simulink model "SnapshotPlanner"  (R2024b)
settings: Solver=FixedStepAuto  StartTime=0.0  StopTime=10.0  RelTol=1e-3  EnableMultiTasking=on
values from neighbouring files (symbols this model uses):
  timeResolution = 0.1    [helperSLHighwayLaneChangePlannerSetup.m]
undefined symbols (not defined in the file or in its folder): actorProfiles, computeMethod
settings Model: Creator=The MathWorks, Inc.  LastModifiedBy=grape
settings SolverCC: AlgebraicLoopSolver=TrustRegion  MaxZcPerStep=1
settings DataIOCC: SaveOutput=off
settings OptimizationCC: DefaultParameterBehavior=Inlined  InlineInvariantSignals=on  EnhancedBackFolding=on  PassReuseOutputArgsAs=Individual arguments  ZeroExternalMemoryAtStartup=off  ZeroInternalMemoryAtStartup=off  EfficientFloat2IntCast=on  OptimizeBlockOrder=speed  DifferentSizesBufferReuse=on  OptimizationCustomize=off  EfficientTunableParamExpr=on
settings DebuggingCC: ParameterTunabilityLossMsg=error  UnconnectedInputMsg=warning  UnconnectedOutputMsg=warning  UnconnectedLineMsg=warning  ModelReferenceSymbolNameMessage=none  SubsystemReferenceDiagnosticForUnitTest=warning
settings HardwareCC: ProdLongLongMode=on
settings ModelReferenceCC: EnableRefExpFcnMdlSchedulingChecks=on  ModelReferenceNumInstancesAllowed=Single  PropagateVarSize=During execution
settings RTWCC: Description=Embedded Coder  SystemTargetFile=ert.tlc  TemplateMakefile=ert_default_tmf  RTWVerbose=off  BuildConfiguration=Faster Runs  PortableWordSizes=on  CodeExecutionProfiling=on  CodeProfilingSaveOptions=AllData  TargetLang=C++  GPUComputeCapability=3.5  DLArmComputeVersion=19.05
settings CodeAppCC: ForceParamTrailComments=on  IgnoreCustomStorageClasses=off  OperatorAnnotations=on  SimulinkDataObjDesc=on  SFDataObjDesc=on  CustomSymbolStrGlobalVar=$N$M  CustomSymbolStrType=$N$M_T  CustomSymbolStrFcn=APV_$N$M$F  CustomSymbolStrMacro=$N$M  InsertBlockDesc=on
settings ERTTargetCC: TargetLangStandard=C++03 (ISO)  GenerateSampleERTMain=on  CombineSignalStateStructs=on  CodeInterfacePackaging=C++ class  SupportVariableSizeSignals=on  RootIOFormat=Structure reference  ERTCustomFileTemplate=example_file_process.tlc  DynamicArrayContainerType=coder::array

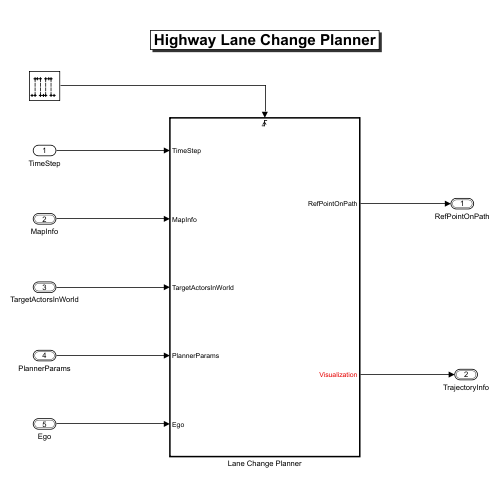
[thumbnail: Simulink's stored preview of the top-level diagram]
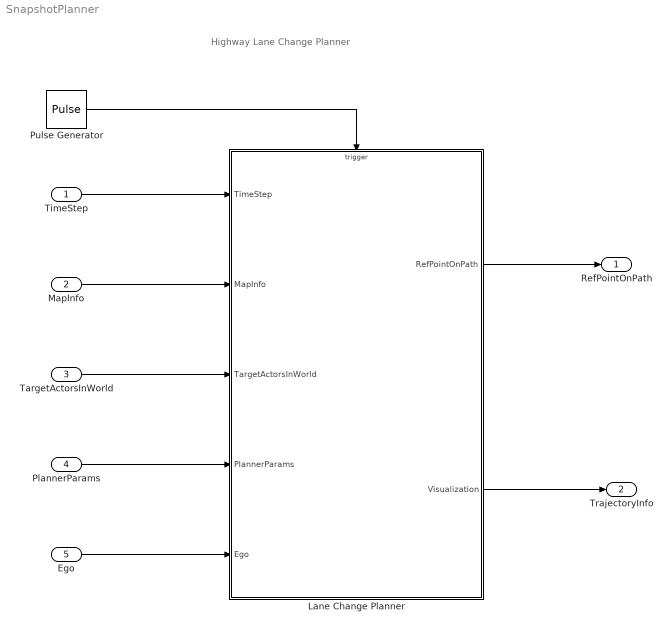
== system SnapshotPlanner ==
  note: Highway Lane Change Planner
  TimeStep : Inport
  MapInfo : Inport  Port=2  OutDataTypeStr=Bus: BusMapInfo  BusOutputAsStruct=on
  TargetActorsInWorld : Inport  Port=3  OutDataTypeStr=Bus: BusActorsEgo  BusOutputAsStruct=on
  PlannerParams : Inport  Port=4  OutDataTypeStr=Bus: BusPlannerParams  BusOutputAsStruct=on
  Ego : Inport  Port=5  OutDataTypeStr=Bus: BusVehiclePose
  Lane Change Planner : Subsystem
  Pulse Generator : DiscretePulseGenerator  SampleTime=timeResolution
  RefPointOnPath : Outport  OutDataTypeStr=Bus: BusRefPointOnPath  BusOutputAsStruct=on
  TrajectoryInfo : Outport  Port=2  OutDataTypeStr=Bus: BusVisualizationInfo  BusOutputAsStruct=on
  wires:
  TimeStep/1 -> Lane Change Planner/1(TimeStep)
  MapInfo/1 -> Lane Change Planner/2(MapInfo)
  TargetActorsInWorld/1 -> Lane Change Planner/3(TargetActorsInWorld)
  PlannerParams/1 -> Lane Change Planner/4(PlannerParams)
  Ego/1 -> Lane Change Planner/5(Ego)
  Lane Change Planner/2(Visualization) -> TrajectoryInfo/1
  Pulse Generator/1 -> Lane Change Planner/Trigger
  Lane Change Planner/1(RefPointOnPath) -> RefPointOnPath/1

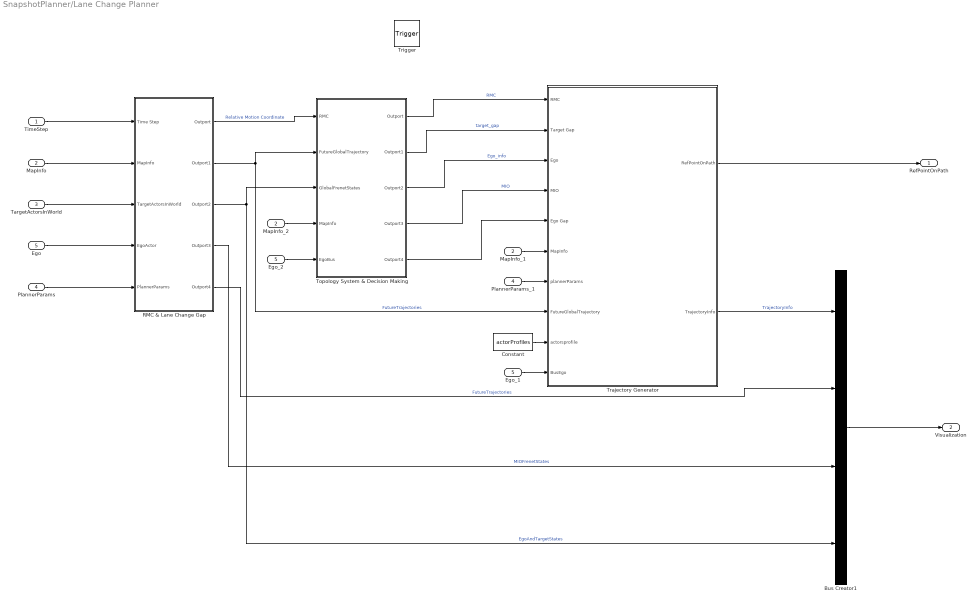
== system SnapshotPlanner/Lane Change Planner ==
  TimeStep : Inport
  MapInfo : Inport  Port=2  OutDataTypeStr=Bus: BusMapInfo  BusOutputAsStruct=on
  TargetActorsInWorld : Inport  Port=3  OutDataTypeStr=Bus: BusActorsEgo  BusOutputAsStruct=on
  PlannerParams : Inport  Port=4  OutDataTypeStr=Bus: BusPlannerParams  BusOutputAsStruct=on
  Ego : Inport  Port=5  OutDataTypeStr=Bus: BusVehiclePose
  Trigger : TriggerPort  VariantControl=(inherit)  InitialTriggerSignalState=zero  PortDimensions=1
  Bus Creator1 : BusCreator  Inputs=4  OutDataTypeStr=Bus: BusVisualizationInfo
  Constant : Constant  Value=actorProfiles  OutDataTypeStr=Bus: BusActorProfiles
  Ego_1 : InportShadow  Port=5  OutDataTypeStr=Bus: BusVehiclePose
  Ego_2 : InportShadow  Port=5  OutDataTypeStr=Bus: BusVehiclePose
  MapInfo_1 : InportShadow  Port=2  OutDataTypeStr=Bus: BusMapInfo  BusOutputAsStruct=on
  MapInfo_2 : InportShadow  Port=2  OutDataTypeStr=Bus: BusMapInfo  BusOutputAsStruct=on
  PlannerParams_1 : InportShadow  Port=4  OutDataTypeStr=Bus: BusPlannerParams  BusOutputAsStruct=on
  "RMC & Lane Change Gap " : Subsystem
  Topology System & Decision Making : Subsystem
  Trajectory Generator : Subsystem
  RefPointOnPath : Outport  OutDataTypeStr=Bus: BusRefPointOnPath  BusOutputAsStruct=on
  Visualization : Outport  Port=2  OutDataTypeStr=Bus: BusVisualizationInfo  BusOutputAsStruct=on
  wires:
  "RMC & Lane Change Gap "/5(Outport4) -> Bus Creator1/2  "FutureTrajectories"
  MapInfo_2/1 -> Topology System & Decision Making/4(MapInfo)
  "RMC & Lane Change Gap "/3(Outport2) -> Bus Creator1/4, Topology System & Decision Making/3(GlobalFrenetStates)  "EgoAndTargetStates"
  "RMC & Lane Change Gap "/1(Outport) -> Topology System & Decision Making/1(RMC)  "Relative Motion Coordinate"
  Topology System & Decision Making/5(Outport4) -> Trajectory Generator/5(Ego Gap)
  Topology System & Decision Making/4(Outport3) -> Trajectory Generator/4(MIO)  "MIO"
  Ego/1 -> "RMC & Lane Change Gap "/4(EgoActor)
  Ego_1/1 -> Trajectory Generator/10(BusEgo)
  "RMC & Lane Change Gap "/2(Outport1) -> Trajectory Generator/8(FutureGlobalTrajectory), Topology System & Decision Making/2(FutureGlobalTrajectory)  "FutureTrajectories"
  PlannerParams/1 -> "RMC & Lane Change Gap "/5(PlannerParams)
  Trajectory Generator/2(TrajectoryInfo) -> Bus Creator1/1  "TrajectoryInfo"
  TimeStep/1 -> "RMC & Lane Change Gap "/1(Time Step)
  TargetActorsInWorld/1 -> "RMC & Lane Change Gap "/3(TargetActorsInWorld)
  Topology System & Decision Making/1(Outport) -> Trajectory Generator/1(RMC)  "RMC"
  Topology System & Decision Making/2(Outport1) -> Trajectory Generator/2(Target Gap)  "target_gap"
  PlannerParams_1/1 -> Trajectory Generator/7(plannerParams)
  MapInfo_1/1 -> Trajectory Generator/6(MapInfo)
  Constant/1 -> Trajectory Generator/9(actorsprofile)
  Topology System & Decision Making/3(Outport2) -> Trajectory Generator/3(Ego)  "Ego_info"
  MapInfo/1 -> "RMC & Lane Change Gap "/2(MapInfo)
  Bus Creator1/1 -> Visualization/1
  "RMC & Lane Change Gap "/4(Outport3) -> Bus Creator1/3  "MIOFrenetStates"
  Ego_2/1 -> Topology System & Decision Making/5(EgoBus)
  Trajectory Generator/1(RefPointOnPath) -> RefPointOnPath/1

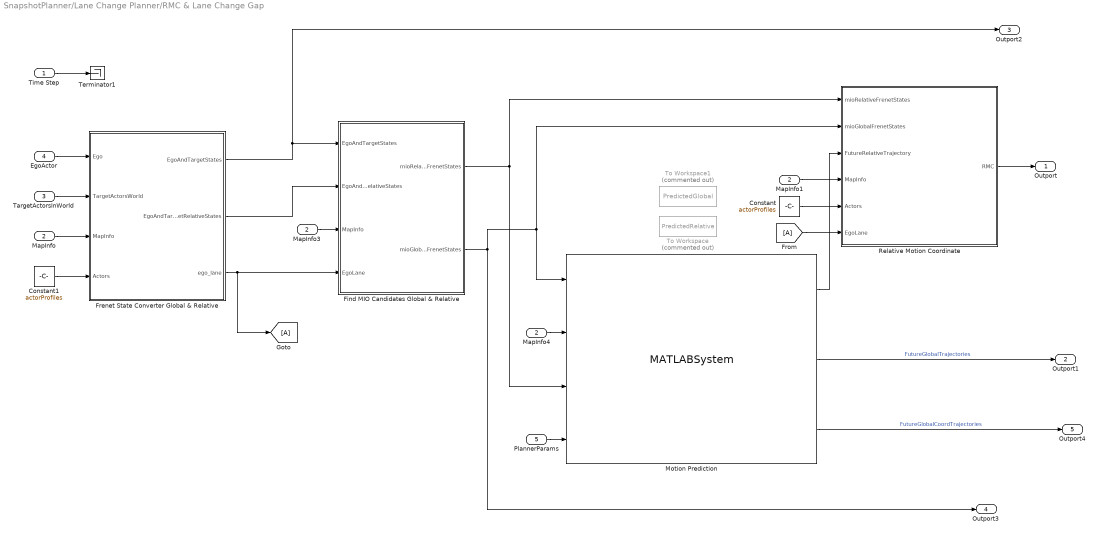
== system SnapshotPlanner/Lane Change Planner/RMC & Lane Change Gap  ==
  Time Step : Inport
  MapInfo : Inport  Port=2  OutDataTypeStr=Bus: BusMapInfo
  TargetActorsInWorld : Inport  Port=3  OutDataTypeStr=Bus: BusActorsEgo
  EgoActor : Inport  Port=4  OutDataTypeStr=Bus: BusVehiclePose
  PlannerParams : Inport  Port=5  OutDataTypeStr=Bus: BusPlannerParams
  Constant : Constant  Value=actorProfiles  OutDataTypeStr=Bus: BusActorProfiles
  Constant1 : Constant  Value=actorProfiles  OutDataTypeStr=Bus: BusActorProfiles
  Find MIO Candidates Global & Relative : MATLAB Function  TreatAsAtomicUnit=on
  Frenet State Converter Global & Relative : MATLAB Function  TreatAsAtomicUnit=on
  From : From
  Goto : Goto
  MapInfo1 : InportShadow  Port=2  OutDataTypeStr=Bus: BusMapInfo
  MapInfo3 : InportShadow  Port=2  OutDataTypeStr=Bus: BusMapInfo
  MapInfo4 : InportShadow  Port=2  OutDataTypeStr=Bus: BusMapInfo
  Motion Prediction : MATLABSystem  System=HelperMotionPrediction_RMC  SimulateUsing=Interpreted execution
      mask Type: HelperMotionPrediction_RMC
      mask Display:
      | disp('HelperMotionPrediction_RMC');
      | port_label('input',1,'MIOs_Global');
      | port_label('input',2,'MapInfo');
      | port_label('input',3,'MIOs_Relative');
      | port_label('input',4,'Params');
      | port_label('output',1,'FutureRelativeTrajectories');
      | port_label('output',2,'FutureGlobalTrajectories');
      | port_label('output',3,'FutureGlobalCoordTrajectories');
  Relative Motion Coordinate : MATLAB Function  TreatAsAtomicUnit=on
  Terminator1 : Terminator
  To Workspace : ToWorkspace  Commented=on  VariableName=PredictedRelative  SaveFormat=Timeseries  SampleTime=-1
  To Workspace1 : ToWorkspace  Commented=on  VariableName=PredictedGlobal  SaveFormat=Timeseries  SampleTime=-1
  Outport : Outport  OutDataTypeStr=Bus: BusRelativeMotionCoordinate
  Outport1 : Outport  Port=2  OutDataTypeStr=Bus: BusPredictedTrajectories
  Outport2 : Outport  Port=3  OutDataTypeStr=Bus: BusEgoAndTargetStates
  Outport3 : Outport  Port=4  OutDataTypeStr=Bus: BusMIOFrenetStates
  Outport4 : Outport  Port=5
  wires:
  Frenet State Converter Global & Relative/1(EgoAndTargetStates) -> Outport2/1, Find MIO Candidates Global & Relative/1(EgoAndTargetStates)
  Time Step/1 -> Terminator1/1
  EgoActor/1 -> Frenet State Converter Global & Relative/1(Ego)
  TargetActorsInWorld/1 -> Frenet State Converter Global & Relative/2(TargetActorsWorld)
  MapInfo/1 -> Frenet State Converter Global & Relative/3(MapInfo)
  Frenet State Converter Global & Relative/2(EgoAndTargetRelativeStates) -> Find MIO Candidates Global & Relative/2(EgoAndTargetRelativeStates)
  MapInfo3/1 -> Find MIO Candidates Global & Relative/3(MapInfo)
  Find MIO Candidates Global & Relative/1(mioRelativeFrenetStates) -> Relative Motion Coordinate/1(mioRelativeFrenetStates), Motion Prediction/3
  MapInfo4/1 -> Motion Prediction/2
  PlannerParams/1 -> Motion Prediction/4
  Find MIO Candidates Global & Relative/2(mioGlobalFrenetStates) -> Relative Motion Coordinate/2(mioGlobalFrenetStates), Motion Prediction/1, Outport3/1
  Motion Prediction/1 -> Relative Motion Coordinate/3(FutureRelativeTrajectory)
  Relative Motion Coordinate/1(RMC) -> Outport/1
  Motion Prediction/2 -> Outport1/1  "FutureGlobalTrajectories"
  MapInfo1/1 -> Relative Motion Coordinate/4(MapInfo)
  Constant/1 -> Relative Motion Coordinate/5(Actors)
  Motion Prediction/3 -> Outport4/1  "FutureGlobalCoordTrajectories"
  Constant1/1 -> Frenet State Converter Global & Relative/4(Actors)
  Frenet State Converter Global & Relative/3(ego_lane) -> Find MIO Candidates Global & Relative/4(EgoLane), Goto/1
  From/1 -> Relative Motion Coordinate/6(EgoLane)

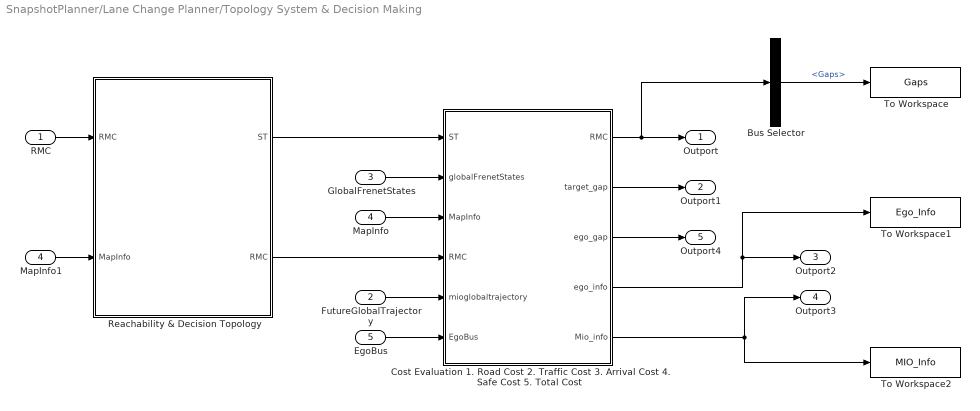
== system SnapshotPlanner/Lane Change Planner/Topology System & Decision Making ==
  RMC : Inport  OutDataTypeStr=Bus: BusRelativeMotionCoordinate
  FutureGlobalTrajectory : Inport  Port=2
  GlobalFrenetStates : Inport  Port=3  OutDataTypeStr=Bus: BusEgoAndTargetStates
  MapInfo : Inport  Port=4
  EgoBus : Inport  Port=5
  Bus Selector : BusSelector  OutputSignals=Gaps
  Cost Evaluation 1. Road Cost 2. Traffic Cost 3. Arrival Cost 4. Safe Cost 5. Total Cost : MATLAB Function  TreatAsAtomicUnit=on
  MapInfo1 : InportShadow  Port=4
  Reachability & Decision Topology : MATLAB Function  TreatAsAtomicUnit=on
  To Workspace : ToWorkspace  VariableName=Gaps  SaveFormat=Timeseries  SampleTime=-1
  To Workspace1 : ToWorkspace  VariableName=Ego_Info  SampleTime=-1
  To Workspace2 : ToWorkspace  VariableName=MIO_Info  SampleTime=-1
  Outport : Outport
  Outport1 : Outport  Port=2
  Outport2 : Outport  Port=3
  Outport3 : Outport  Port=4
  Outport4 : Outport  Port=5
  wires:
  Reachability & Decision Topology/2(RMC) -> Cost Evaluation 1. Road Cost 2. Traffic Cost 3. Arrival Cost 4. Safe Cost 5. Total Cost/4("RMC ")
  Reachability & Decision Topology/1(ST) -> Cost Evaluation 1. Road Cost 2. Traffic Cost 3. Arrival Cost 4. Safe Cost 5. Total Cost/1(ST)
  MapInfo/1 -> Cost Evaluation 1. Road Cost 2. Traffic Cost 3. Arrival Cost 4. Safe Cost 5. Total Cost/3(MapInfo)
  FutureGlobalTrajectory/1 -> Cost Evaluation 1. Road Cost 2. Traffic Cost 3. Arrival Cost 4. Safe Cost 5. Total Cost/5(mioglobaltrajectory)
  RMC/1 -> Reachability & Decision Topology/1("RMC ")
  GlobalFrenetStates/1 -> Cost Evaluation 1. Road Cost 2. Traffic Cost 3. Arrival Cost 4. Safe Cost 5. Total Cost/2(globalFrenetStates)
  Cost Evaluation 1. Road Cost 2. Traffic Cost 3. Arrival Cost 4. Safe Cost 5. Total Cost/1(RMC) -> Bus Selector/1, Outport/1
  Cost Evaluation 1. Road Cost 2. Traffic Cost 3. Arrival Cost 4. Safe Cost 5. Total Cost/4(ego_info) -> To Workspace1/1, Outport2/1
  Cost Evaluation 1. Road Cost 2. Traffic Cost 3. Arrival Cost 4. Safe Cost 5. Total Cost/2(target_gap) -> Outport1/1
  Cost Evaluation 1. Road Cost 2. Traffic Cost 3. Arrival Cost 4. Safe Cost 5. Total Cost/5(Mio_info) -> Outport3/1, To Workspace2/1
  Cost Evaluation 1. Road Cost 2. Traffic Cost 3. Arrival Cost 4. Safe Cost 5. Total Cost/3(ego_gap) -> Outport4/1
  Bus Selector/1 -> To Workspace/1  "<Gaps>"
  MapInfo1/1 -> Reachability & Decision Topology/2(MapInfo)
  EgoBus/1 -> Cost Evaluation 1. Road Cost 2. Traffic Cost 3. Arrival Cost 4. Safe Cost 5. Total Cost/6(EgoBus)

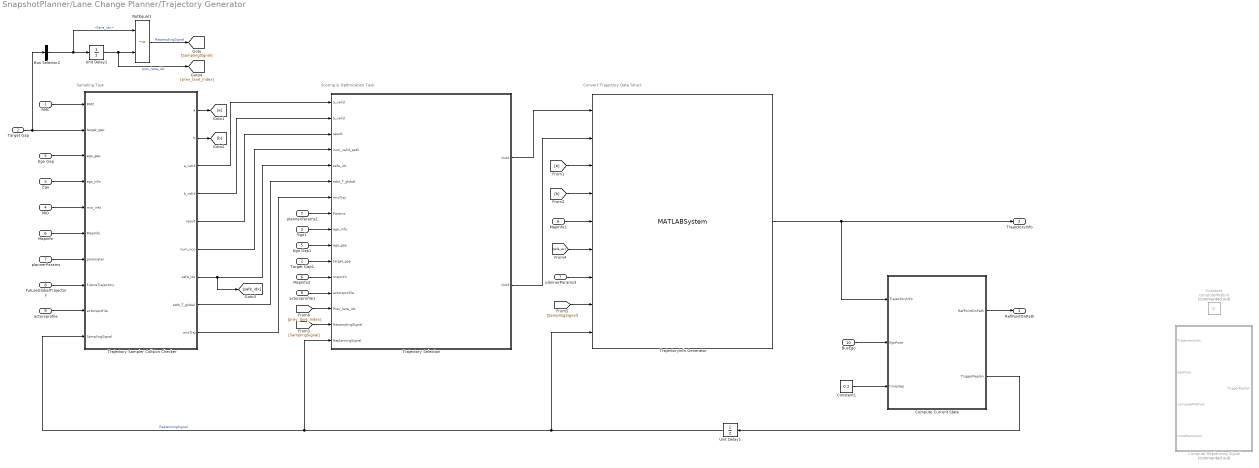
== system SnapshotPlanner/Lane Change Planner/Trajectory Generator ==
  note: Convert Trajectory Data Struct
  note: Scoring & Optimization Task
  note: Sampling Task
  RMC : Inport  OutDataTypeStr=Bus: BusRelativeMotionCoordinate
  Target Gap : Inport  Port=2
  Ego : Inport  Port=3
  MIO : Inport  Port=4
  Ego Gap : Inport  Port=5
  MapInfo : Inport  Port=6
  plannerParams : Inport  Port=7
  FutureGlobalTrajectory : Inport  Port=8
  actorsprofile : Inport  Port=9
  BusEgo : Inport  Port=10  OutDataTypeStr=Bus: BusVehiclePose
  Bus Selector2 : BusSelector  OutputSignals=lane_idx
  Compute Current State : MATLAB Function  TreatAsAtomicUnit=on
  Compute Replanning Signal : MATLAB Function  Commented=on  TreatAsAtomicUnit=on
  Constant : Constant  Commented=on  Value=computeMethod
  Constant1 : Constant  Value=0.2
  Ego Gap1 : InportShadow  Port=5
  Ego1 : InportShadow  Port=3
  MapInfo1 : InportShadow  Port=6
  MapInfo2 : InportShadow  Port=6
  NotEqual1 : RelationalOperator  Operator=~=  OutDataTypeStr=boolean  RndMeth=Simplest  InputSameDT=off
  Target Gap1 : InportShadow  Port=2
  Trajectory Selection : Subsystem  TreatAsAtomicUnit=on
  Trajectory Sampler Collsion Checker : MATLAB Function  TreatAsAtomicUnit=on
  TrajectoryInfo Generator : MATLABSystem  System=HelperMakeTrajectoryInfo  SimulateUsing=Interpreted execution
      mask Type: HelperMakeTrajectoryInfo
      mask Display:
      | disp('HelperMakeTrajectoryInfo');
      | port_label('input',1,'optimal_a');
      | port_label('input',2,'optimal_b');
      | port_label('input',3,'a');
      | port_label('input',4,'b');
      | port_label('input',5,'MapInfo');
      | port_label('input',6,'safe_idx');
      | port_label('input',7,'params');
      | port_label('input',8,'resamplingSignal');
      | port_label('input',9,'replanningSignal');
      | port_label('output',1,'GlobalTrajectories');
  Unit Delay1 : UnitDelay  InitialCondition=true  SampleTime=-1  HasFrameUpgradeWarning=on
  Unit Delay2 : UnitDelay  SampleTime=-1  HasFrameUpgradeWarning=on
  actorsprofile1 : InportShadow  Port=9
  plannerParams1 : InportShadow  Port=7
  plannerParams3 : InportShadow  Port=7
  RefPointOnPath : Outport  OutDataTypeStr=Bus: BusRefPointOnPath
  TrajectoryInfo : Outport  Port=2  OutDataTypeStr=Bus: BusGlobalTrajectories
  wires:
  MapInfo/1 -> Trajectory Sampler Collsion Checker/6(MapInfo)
  Ego/1 -> Trajectory Sampler Collsion Checker/4(ego_info)
  RMC/1 -> Trajectory Sampler Collsion Checker/1(RMC)
  MIO/1 -> Trajectory Sampler Collsion Checker/5(mio_info)
  plannerParams/1 -> Trajectory Sampler Collsion Checker/7(parameter)
  FutureGlobalTrajectory/1 -> Trajectory Sampler Collsion Checker/8(FutureTrajectory)
  actorsprofile/1 -> Trajectory Sampler Collsion Checker/9(actorsprofile)
  Ego Gap/1 -> Trajectory Sampler Collsion Checker/3(ego_gap)
  TrajectoryInfo Generator/1 -> Compute Current State/1(TrajectoryInfo), TrajectoryInfo/1
  Bus Selector2/1 -> NotEqual1/1, Unit Delay2/1  "<lane_idx>"
  Unit Delay2/1 -> [prev_lane_index], NotEqual1/2  "prev_lane_idx"
  Target Gap/1 -> Bus Selector2/1, Trajectory Sampler Collsion Checker/2(target_gap)
  Unit Delay1/1 -> Trajectory Sampler Collsion Checker/10(SamplingSignal), Trajectory Selection/16(ReplanningSignal), TrajectoryInfo Generator/9  "ReplanningSignal"
  NotEqual1/1 -> [SamplingSignal]  "ResamplingSignal"
  Trajectory Sampler Collsion Checker/2(b) -> [b]
  Trajectory Sampler Collsion Checker/1(a) -> [a]
  [a] -> TrajectoryInfo Generator/3
  [b] -> TrajectoryInfo Generator/4
  Trajectory Selection/1(Out2) -> TrajectoryInfo Generator/1
  Trajectory Selection/2(Out3) -> TrajectoryInfo Generator/2
  MapInfo1/1 -> TrajectoryInfo Generator/5
  Trajectory Sampler Collsion Checker/3(a_valid) -> Trajectory Selection/1(a_valid)
  Trajectory Sampler Collsion Checker/4(b_valid) -> Trajectory Selection/2(b_valid)
  Trajectory Sampler Collsion Checker/5(result) -> Trajectory Selection/3(result)
  Trajectory Sampler Collsion Checker/6(num_ncp) -> Trajectory Selection/4(num_valid_path)
  Trajectory Sampler Collsion Checker/7(safe_idx) -> [safe_idx], Trajectory Selection/5(safe_idx)
  Trajectory Sampler Collsion Checker/8(sdot_T_global) -> Trajectory Selection/6(sdot_T_global)
  Trajectory Sampler Collsion Checker/9(mioTraj) -> Trajectory Selection/7(mioTraj)
  plannerParams1/1 -> Trajectory Selection/8(Params)
  Ego1/1 -> Trajectory Selection/9(ego_info)
  Ego Gap1/1 -> Trajectory Selection/10(ego_gap)
  Target Gap1/1 -> Trajectory Selection/11(target_gap)
  MapInfo2/1 -> Trajectory Selection/12(mapinfo)
  actorsprofile1/1 -> Trajectory Selection/13(actorsprofile)
  [safe_idx] -> TrajectoryInfo Generator/6
  plannerParams3/1 -> TrajectoryInfo Generator/7
  [SamplingSignal] -> TrajectoryInfo Generator/8
  [SamplingSignal] -> Trajectory Selection/15(ResamplingSignal)
  [prev_lane_index] -> Trajectory Selection/14(Prev_lane_idx)
  Compute Current State/2(TriggerReplan) -> Unit Delay1/1
  BusEgo/1 -> Compute Current State/2(EgoPose)
  Constant1/1 -> Compute Current State/3(timestep)
  Compute Current State/1(RefPointOnPath) -> RefPointOnPath/1

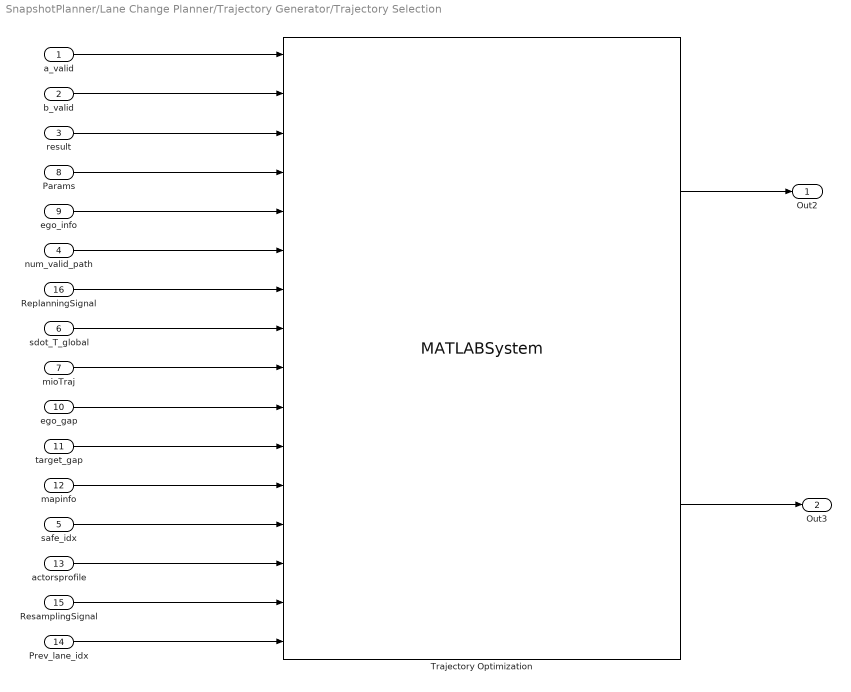
== system SnapshotPlanner/Lane Change Planner/Trajectory Generator/Trajectory Selection ==
  a_valid : Inport
  b_valid : Inport  Port=2
  result : Inport  Port=3
  num_valid_path : Inport  Port=4
  safe_idx : Inport  Port=5
  sdot_T_global : Inport  Port=6
  mioTraj : Inport  Port=7
  Params : Inport  Port=8
  ego_info : Inport  Port=9
  ego_gap : Inport  Port=10
  target_gap : Inport  Port=11
  mapinfo : Inport  Port=12
  actorsprofile : Inport  Port=13
  Prev_lane_idx : Inport  Port=14
  ResamplingSignal : Inport  Port=15
  ReplanningSignal : Inport  Port=16
  Trajectory Optimization : MATLABSystem  System=HelperSelectionTrajectory  SimulateUsing=Interpreted execution
      mask Type: HelperSelectionTrajectory
      mask Display:
      | disp('HelperSelectionTrajectory');
      | port_label('input',1,'a_valid');
      | port_label('input',2,'b_valid');
      | port_label('input',3,'result');
      | port_label('input',4,'Params');
      | port_label('input',5,'ego_info');
      | port_label('input',6,'num_valid_path');
      | port_label('input',7,'replanningSignal');
      | port_label('input',8,'sdot_T_global');
      | port_label('input',9,'mioTraj');
      | port_label('input',10,'ego_gap');
      | port_label('input',11,'target_gap');
      | port_label('input',12,'mapInfo');
      | port_label('input',13,'safe_idx');
      | port_label('input',14,'actorsprofile');
      | port_label('input',15,'resamplingSignal');
      | port_label('input',16,'Prev_lane_idx');
      | port_label('output',1,'optimal_a');
      | port_label('output',2,'optimal_b');
  Out2 : Outport
  Out3 : Outport  Port=2
  wires:
  Params/1 -> Trajectory Optimization/4
  actorsprofile/1 -> Trajectory Optimization/14
  ego_info/1 -> Trajectory Optimization/5
  sdot_T_global/1 -> Trajectory Optimization/8
  mapinfo/1 -> Trajectory Optimization/12
  b_valid/1 -> Trajectory Optimization/2
  ReplanningSignal/1 -> Trajectory Optimization/7
  safe_idx/1 -> Trajectory Optimization/13
  mioTraj/1 -> Trajectory Optimization/9
  target_gap/1 -> Trajectory Optimization/11
  a_valid/1 -> Trajectory Optimization/1
  Trajectory Optimization/1 -> Out2/1
  result/1 -> Trajectory Optimization/3
  num_valid_path/1 -> Trajectory Optimization/6
  ego_gap/1 -> Trajectory Optimization/10
  Trajectory Optimization/2 -> Out3/1
  ResamplingSignal/1 -> Trajectory Optimization/15
  Prev_lane_idx/1 -> Trajectory Optimization/16

== matlab function SnapshotPlanner/Lane Change Planner/RMC & Lane Change Gap /Frenet State Converter Global & Relative ==
  data: EgoAndTargetStates output Bus: BusEgoAndTargetStates; Ego input; TargetActorsWorld input; MapInfo input; EgoAndTargetRelativeStates output Bus: BusEgoAndTargetRelativeStates; Actors input; ego_lane output
function [EgoAndTargetStates, EgoAndTargetRelativeStates, ego_lane] = frenetStateConverter(Ego,... 
                                                                                 TargetActorsWorld,...
                                                                                 MapInfo, Actors)
                                                   
coder.inline('never');
persistent RefPathFrenet

% Load all actor's path points
refPath = MapInfo.GlobalPlanPoints(1:MapInfo.NumGlobalPlanPoints,:);


if isempty(RefPathFrenet)
    % Initialization : GlobalWaypoints
    RefPathFrenet = referencePathFrenet(refPath);   
else
    % Check for a change in the reference path
    if ~isequal(RefPathFrenet.Waypoints, refPath) 
        refPathNew = referencePathFrenet(refPath);
        RefPathFrenet.Waypoints = refPathNew.Waypoints;
    end
end

% Initialize output bus
egoAndTargetStates = HelperLCPlannerDefaultData.EgoAndTargetStates;
egoAndTargetRelativeStates = HelperLCPlannerDefaultData.EgoAndTargetRelativeStates;


kapa = deg2rad(Ego.AngularVelocity(3))/norm(Ego.Velocity);
if (isnan(kapa) || isinf(kapa))
    kapa = 0;
end
egoState = [Ego.Position(1:2), deg2rad(Ego.Yaw), kapa, norm(Ego.Velocity(1:2),2), norm(Ego.Acceleration(1:2), 2)];%Update the acceleration state

% Frenet States : [x, y, theta, kappa, velocity, acceleration]
% global2frenet : internal function
egoFrenetState = global2frenet(RefPathFrenet, egoState);
targetStates = zeros(TargetActorsWorld.NumActors, 6);
numTargets = TargetActorsWorld.NumActors;
targetFrenetStates = zeros(numTargets, 6);
targetIDs = zeros(numTargets,1);

targetRelativeStates = zeros(numTargets, 6);
targetRelativeFrenetStates = zeros(numTargets, 6);

for i=1:numTargets
    vel = norm(TargetActorsWorld.Actors(i).Velocity(1:2));
    kappa = deg2rad(TargetActorsWorld.Actors(i).AngularVelocity(3))/vel;
    if (isnan(kappa) || isinf(kappa))
        kappa = 0;
    end

    targetStates(i,:) = [TargetActorsWorld.Actors(i).Position(1:2),...
                       deg2rad(TargetActorsWorld.Actors(i).Yaw), kappa,...
                       vel, 0];

    targetIDs(i,1) = TargetActorsWorld.Actors(i).ActorID;
    targetFrenetStates(i,:) = global2frenet(RefPathFrenet, targetStates(i,:));

    targetRelativeStates(i, :) = targetStates(i, :) - egoState;

    targetRelativeFrenetStates(i, 1) = targetFrenetStates(i, 1) - egoFrenetState(1); % s
    targetRelativeFrenetStates(i, 2) = targetFrenetStates(i, 2) - egoFrenetState(2); % ds
    targetRelativeFrenetStates(i, 3) = targetFrenetStates(i, 3) - egoFrenetState(3); % dds
    targetRelativeFrenetStates(i, 4) = targetFrenetStates(i, 4) - egoFrenetState(4); % l
    targetRelativeFrenetStates(i, 5) = targetFrenetStates(i, 5) - egoFrenetState(5); % dl
    targetRelativeFrenetStates(i, 6) = targetFrenetStates(i, 6) - egoFrenetState(6); % ddl 


    % Update the lateral and logitudinal  frenet states to zero when the
    % speed is zero.
    if abs(targetStates(i,5)) < 1e-3
        targetFrenetStates(i,2) = 0;
        targetFrenetStates(i,5) = 0;

    end
end

egoAndTargetStates.NumTargetActors = numTargets;
egoAndTargetStates.TargetGlobalStates(1:numTargets,:) = targetStates;
egoAndTargetStates.TargetFrenetStates(1:numTargets,:) = targetFrenetStates;
egoAndTargetStates.TargetIDs(1:numTargets,:) = targetIDs;
egoAndTargetStates.EgoGlobalState = egoState;
egoAndTargetStates.EgoFrenetState = egoFrenetState;
EgoAndTargetStates = egoAndTargetStates;

egoAndTargetRelativeStates.NumTargetActors = numTargets;
egoAndTargetRelativeStates.TargetRelativeStates(1:numTargets,:) = targetRelativeStates;
egoAndTargetRelativeStates.TargetRelativeFrenetStates(1:numTargets,:) = targetRelativeFrenetStates;
egoAndTargetRelativeStates.TargetIDs(1:numTargets,:) = targetIDs;
egoAndTargetRelativeStates.EgoGlobalFrenetState = egoFrenetState;
EgoAndTargetRelativeStates = egoAndTargetRelativeStates;


%%%%%%%%%%%%%%%% Ego 차량 자체의 차선 판단은 보수적으로.. %%%%%%%%%%%%%%%%%%

ego_length = Actors(1).Length;
ego_width = Actors(1).Width;
ego_frenet = [egoFrenetState(1); egoFrenetState(4)];
ego_frenet_yaw = rad2deg(atan2(egoFrenetState(5), egoFrenetState(2)));
if abs(ego_frenet_yaw) < 1e-5
    ego_frenet_yaw = 0;
end
rotationMatrix = [cosd(ego_frenet_yaw), -sind(ego_frenet_yaw); sind(ego_frenet_yaw), cosd(ego_frenet_yaw)];

if ego_frenet_yaw > 0
    ego_front_left = rotationMatrix * [ego_length/2; ego_width/2] + ego_frenet;
    ego_lane = helperDetectLaneNumber(MapInfo, ego_front_left(2));
elseif ego_frenet_yaw < 0
    ego_front_right = rotationMatrix * [ego_length/2; -ego_width/2] + ego_frenet;
    ego_lane = helperDetectLaneNumber(MapInfo, ego_front_right(2));
else
    ego_lane = helperDetectLaneNumber(MapInfo, egoFrenetState(4));
end

%%%%%%%%%%% 차선 변경 차량에 대한 Prediction 에서는 이와 반대로 %%%%%%%%%%%%

end

== matlab function SnapshotPlanner/Lane Change Planner/RMC & Lane Change Gap /Relative Motion Coordinate ==
  data: mioRelativeFrenetStates input; mioGlobalFrenetStates input; RMC output Bus: BusRelativeMotionCoordinate; FutureRelativeTrajectory input; MapInfo input; Actors input; EgoLane input
function RMC = MakeRMC(mioRelativeFrenetStates, mioGlobalFrenetStates, FutureRelativeTrajectory, MapInfo, Actors, EgoLane)

%%% mioRelativeFrenetStates %%%
%%% 1. NumMIOs      : MIO 개수
%%% 2. TargetIds    : MIO 차량들의 고유번호
%%% 3. MIOStates    : MIO 차량들의 Frenet States (s ds dds l dl ddl)

%%% FutureRelativeTrajectory %%%
%%% 1. NumTrajs     : Trajectroy 개수 (= MIO 개수)
%%% 2. TargetIDs    : MIO 고유번호
%%% 3. Trajectories : Trajectory 객체 (TargetID, NumPts, Trajectory)

%%% MapInfo %%%
%%% 1. NumLanes             : 차선 개수
%%% 2. LaneWidth            : 차선 폭
%%% 3. LaneCenter           : 차선 중심
%%% 4. NumGlobalPlanPoints  : Global Waypoint 개수
%%% 5. GlobalPlanPoints     : Global Waypoint 초기경로
%%% 6. LaneLateralBoundary  : 차선의 횡방향 Boundary

initStruct = HelperLCPlannerDefaultData.RelativeMotionCoordinate;

% Filter TargetActors to include only those whose ActorID matches the TargetIds in mioRelativeFrenetStates
TargetIds = mioRelativeFrenetStates.TargetIds;
TargetActors = Actors(ismember([Actors.ActorID], TargetIds));
EgoActor = Actors(1); 

RMC = helperCreateRelativeMotionCoordinate(mioRelativeFrenetStates, ...
                                           mioGlobalFrenetStates, ...
                                           FutureRelativeTrajectory, ...
                                           MapInfo, ...
                                           initStruct, ...
                                           TargetActors, ...
                                           EgoActor, EgoLane);

end

== matlab function SnapshotPlanner/Lane Change Planner/RMC & Lane Change Gap /Find MIO Candidates Global & Relative ==
  data: EgoAndTargetStates input; EgoAndTargetRelativeStates input; MapInfo input; mioRelativeFrenetStates output Bus: BusMIOFrenetStates; mioGlobalFrenetStates output Bus: BusMIOFrenetStates; EgoLane input
function [mioRelativeFrenetStates,mioGlobalFrenetStates] =  findMIOs(EgoAndTargetStates,...
                                                                     EgoAndTargetRelativeStates,...
                                                                     MapInfo, EgoLane)

%%% EgoAndTargetRelativeState %%%
%%% 1. NumTargetActors      : 총 주변 차량 수
%%% 2. TargetRelativeStates : 주변 차량의 RelativeStates with respect to World Coordinate(x, y, Yaw, Kappa, Velocity, accel)
%%% 3. TargetFrenetStates   : 주변 차량의 RelativeStates with respect to Frenet States (s, ds, dds, l, dl, ddl)
%%% 4. TargetIDs            : 주변 차량의 고유번호
%%% 5. EgoGlobalFrenetState : Ego 차량의 Frenet States

coder.inline('never');
%findMIOs function block identifies Most Importent Objects(MIOs) in the
%scenario.


% Get the number of target actors in the scenario from EgoAndTargetStates
% bus structure 
numTargets = EgoAndTargetRelativeStates.NumTargetActors;

% Get target actors frenet states from EgoAndTargetStates bus structure.
targetRelativeFrenetStates = EgoAndTargetRelativeStates.TargetRelativeFrenetStates;
targetGlobalFrenetStates = EgoAndTargetStates.TargetFrenetStates;
targetIDs = EgoAndTargetRelativeStates.TargetIDs;

% Get ego actor frenet states from EgoAndTargetStates bus structure
egoFrenetState = EgoAndTargetRelativeStates.EgoGlobalFrenetState;

% Invoke the wrapper function helperFindMIOs to get the MIOs and lead
% vehicle information.
% {NumMios, LaneNumbers, TTc, RelativeDist, RelativeVel, Issafe, Isfront}
initStruct = HelperLCPlannerDefaultData.MIOFrenetStates;
mioRelativeFrenetStates = initStruct;
mioGlobalFrenetStates = initStruct;

% Invoke the wrapper function helperFindMGlobalFrenetStatIOs to get the MIOs and lead
% vehicle information.
if(numTargets)
    [mioRelativeFrenetStates,...
     mioGlobalFrenetStates] =  helperFindMIOCandidates_RMC(egoFrenetState,...
                                                            MapInfo,...
                                                            targetRelativeFrenetStates(1:numTargets,:),...
                                                            targetGlobalFrenetStates(1:numTargets,:),...
                                                            targetIDs(1:numTargets,:), EgoLane, ...
                                                            initStruct);
end

end

== matlab function SnapshotPlanner/Lane Change Planner/Trajectory Generator/Trajectory Sampler Collsion Checker ==
  data: a output; b output; RMC input; a_valid output; target_gap input; ego_gap input; ego_info input; mio_info input; MapInfo input; parameter input; b_valid output; FutureTrajectory input; actorsprofile input; result output; num_ncp output; safe_idx output; SamplingSignal input; sdot_T_global output; mioTraj output Bus: BusMIOInfo
function [a, b, a_valid, b_valid, result, num_ncp, safe_idx, sdot_T_global, mioTraj] = TrajectorySampler(RMC, target_gap, ego_gap, ego_info, mio_info, MapInfo,...
                                                                                           parameter, FutureTrajectory, actorsprofile, SamplingSignal)

    %%% Trajectory Sampling in Global frenet Coordinate %%%
    
    %%% EgoInfo : [s ds l dl Id(=0)]
    %%% mio_info = [s ds d Id lane];
    
    persistent prev_a prev_b prev_a_valid prev_b_valid prev_result prev_num_ncp prev_not_collision_path prev_mioTraj prev_sdot_T_global InitialSpeed
    
    if isempty(prev_a)
        prev_a = zeros(6, 6);
        prev_b = zeros(5, 6);
        prev_a_valid = zeros(6, 6);
        prev_b_valid = zeros(5, 6);
        prev_result = true;
        prev_num_ncp = 6;
        prev_not_collision_path = zeros(1, 6);
        prev_mioTraj = HelperLCPlannerDefaultData.MIOInfo();
        prev_sdot_T_global = 0;
        InitialSpeed = 20;
    end
    
    if SamplingSignal
        a = zeros(6, 6);
        b = zeros(5, 6);
        a_valid= zeros(6, 6);
        b_valid = zeros(5, 6);
        v_limit = 100/3.6;
        a_limit = 3.0;
        
        Gaps = RMC.Gaps;
        numGaps = RMC.NumGaps;
        numMIOs = sum(RMC.veh_number);
        validGaps = Gaps(1:numGaps);
    
    
    %%%%%%%%%%%%%%%%%%%%%% Plotting Behavior Type Cost %%%%%%%%%%%%%%%%%%%%%%%%
    
        % road_cost = [validGaps.road_cost];
        % traffic_cost = [validGaps.traffic_cost];
        % arrival_cost = [validGaps.arrival_cost];
        % total_cost = [validGaps.total_cost];
    
        % figure(5)
        % bar([road_cost; traffic_cost; arrival_cost; total_cost]', 'grouped');
        % legend({'Road Cost', 'Traffic Cost', 'Arrival Cost', 'Total Cost'}, 'Location', 'Best');
        % xlabel('Gap Index');
        % ylabel('Cost Value');
        % title('Comparison of Costs Across Gaps');
    
    %%%%%%%%%%%%%%%%%%%%%%%%%%%%%%%%%%%%%%%%%%%%%%%%%%%%%%%%%%%%%%%%%%%%%%%%%%%
    
        if numMIOs == 0
            mio_s = 0;
            mio_vel = 0;
            mio_lane = 0;
            mio_traj = FutureTrajectory;
        else
            mio_s = mio_info(1, 1:numMIOs);
            mio_vel = mio_info(2, 1:numMIOs);
            mio_lane = mio_info(end, 1:numMIOs);
            mio_traj = FutureTrajectory;
        end
        
        target_lane = target_gap.lane_idx;
        ego_lane = ego_gap.lane_idx;
        d_target = target_gap.d;
        ego_s = ego_info(1); % s
        ego_vel = ego_info(2); % ds
        ego_acc = ego_info(3);
    
        %% Boundary Conditions for Velocity Planning
        if target_lane == ego_lane
            if RMC.veh_number(target_lane) == 0
                sdot_T = InitialSpeed;
            else
                mio_ego_lane = find(mio_lane == target_lane);
                mio_ego_lane_front = mio_s(mio_ego_lane) > ego_s;
                if any(mio_ego_lane_front)
                    [~, mio_min] = min(mio_s(mio_ego_lane(mio_ego_lane_front)));
                    mio_min = mio_min(1);
                    sdot_T = mio_vel(mio_ego_lane(mio_min));
                else
                    mio_rear_vel = max(mio_vel(mio_ego_lane));
                    mio_rear_vel = mio_rear_vel(1);
                    if mio_rear_vel > ego_vel
                        sdot_T = mio_rear_vel;
                    else
                        sdot_T = InitialSpeed;
                    end
                end
            end
        else
            if RMC.veh_number(target_lane) == 0
                sdot_T = InitialSpeed;
            else
                mio_target_lane = find(mio_lane == target_lane);
                mio_target_front = mio_s(mio_target_lane) > ego_s;
                if any(mio_target_front)
                    [~, mio_min] = min(mio_s(mio_target_lane(mio_target_front)));
                    mio_min = mio_min(1);
                    sdot_T = mio_vel(mio_target_lane(mio_min));
                else
                    mio_rear_vel = max(mio_vel(mio_target_lane));
                    mio_rear_vel = mio_rear_vel(1);
                    if mio_rear_vel > ego_vel
                        sdot_T = mio_rear_vel;
                    else
                        sdot_T = InitialSpeed;
                    end
                end
            end
        end
        sdot_T_global = sdot_T;
        
        %% Longitudinal Planning
        n = 1;
        s0 = ego_s; % 차량의 질량중심
        v0 = ego_vel; % 차량의 초기속도
        a0 = ego_acc;
        durationTime_sample = length(parameter.TimeHorizon);
        velocity_sample = parameter.velocityHorizon;
        T = parameter.TimeHorizon;
        
        b_0 = s0*ones(1, durationTime_sample*velocity_sample);
        b_1 = v0*ones(1, durationTime_sample*velocity_sample);
        b_2 = 0.5*a0*ones(1, durationTime_sample*velocity_sample);
        b_3 = zeros(1, durationTime_sample*velocity_sample);
        b_4 = zeros(1, durationTime_sample*velocity_sample);
        
        if sdot_T_global ~= v0
            for i = 1:durationTime_sample
                deg = 0;
                while true
                    ds_T = ego_vel + (sdot_T_global - ego_vel) * (0.5)^deg;
                    b3b4 = [3*T(i)^2, 4*T(i)^3; 6*T(i), 12*T(i)^2] \ [ds_T - v0 - a0*T(i) ; 0];
                    b3 = b3b4(1);
                    b4 = b3b4(2);
    
                    max_accel = 2*b_2(n) + 3*b3*T(i) + 3*b4*T(i)^2;
                    % max_accel = GetmaxAccel([b2, b3, b4], T(i));
                    if abs(max_accel) <= a_limit
                        b_3(n) = b3;
                        b_4(n) = b4;
    
                        b3b4_const = [3*T(i)^2, 4*T(i)^3; 6*T(i), 12*T(i)^2] \ [ego_vel - v0 - a0*T(i) ; 0];
                        b_3(n+1) = b3b4_const(1);
                        b_4(n+1) = b3b4_const(2);
                        n = n+2;
                        break;
                    end
    
                    deg = deg+1;
                end
            end 
    
        else
            for i = 1:durationTime_sample
                for j = 1:velocity_sample
                    b3b4 = [3*T(i)^2, 4*T(i)^3; 6*T(i), 12*T(i)^2] \ [ego_vel - v0 - a0*T(i) ; 0];
                    b_3(n) = b3b4(1);
                    b_4(n) = b3b4(2);
                    n = n+1;
                end
            end
        end
        
        %% lateral planning
        n = 1;
        d0  = ego_info(4); % 초기 횡방향 위치
        vd0 = ego_info(5); % 초기 횡방향 속도
        ad0 = ego_info(6); % 초기 횡방향 가속도
        
        a_0 = d0*ones(1, durationTime_sample*velocity_sample);
        a_1 = vd0*ones(1, durationTime_sample*velocity_sample);
        a_2 = 0.5*ad0*ones(1, durationTime_sample*velocity_sample);
        a_3 = zeros(1, durationTime_sample*velocity_sample);
        a_4 = zeros(1, durationTime_sample*velocity_sample);
        a_5 = zeros(1, durationTime_sample*velocity_sample);
        
        for i = 1:durationTime_sample
            for j = 1:velocity_sample
                a3a4a5 = [T(i)^3, T(i)^4, T(i)^5; 3*T(i)^2, 4*T(i)^3, 5*T(i)^4; 6*T(i), 12*T(i)^2, 20*T(i)^3]\...
                         [d_target - d0 - vd0*T(i) - 0.5*ad0*T(i)^2 ; -vd0 - ad0*T(i); -ad0];
    
                a_3(n) = a3a4a5(1);
                a_4(n) = a3a4a5(2);
                a_5(n) = a3a4a5(3);
                n = n+1;
            end
        end
        
        a(1:6, 1:durationTime_sample*velocity_sample) = [a_0;a_1;a_2;a_3;a_4;a_5];
        b(1:5, 1:durationTime_sample*velocity_sample) = [b_0;b_1;b_2;b_3;b_4];
    
    
    
    
        
        %% Collsion Check
        
        [a_valid, b_valid, result, num_ncp, safe_idx, mioTraj] = helperCollisionCheck(RMC, target_gap, ego_gap, mio_info, ego_info, mio_traj, a, b, parameter, actorsprofile);
    
        prev_a = a;
        prev_b = b;
        prev_a_valid = a_valid;
        prev_b_valid = b_valid;
        prev_result = result;
        prev_num_ncp = num_ncp;
        prev_not_collision_path = safe_idx;
        prev_sdot_T_global = sdot_T_global;
        prev_mioTraj = mioTraj;
    
    
    else
        a = prev_a;
        b = prev_b;
        a_valid = prev_a_valid;
        b_valid = prev_b_valid;
        result = prev_result;
        num_ncp = prev_num_ncp;
        safe_idx = prev_not_collision_path;
        mioTraj = prev_mioTraj;
        sdot_T_global = prev_sdot_T_global;
    end

end



function max_accel = GetmaxAccel(coeff, durationtime)
   start_point = durationtime/2;
   criterion = 1e-3;
   learning_rate = 0.001;
   highest_sign = sign(coeff(3));
    
   t = start_point;
   while true
        grad = coeff(2) + 2*coeff(3)*t;

        new_t = t - learning_rate * highest_sign * grad;

        if (abs(new_t - t) / new_t) < criterion
            break;
        else
            t = new_t;
        end
   end
   max_accel = coeff(1) + coeff(2) * t + coeff(3) * t^2;

end

== matlab function SnapshotPlanner/Lane Change Planner/Topology System & Decision Making/Reachability & Decision Topology ==
  data: ST output; RMC input Bus: BusRelativeMotionCoordinate; RMC output; MapInfo input
function [ST, RMC] = ReachableAndTopology(RMC, MapInfo)

Gaps = RMC.Gaps;
x_ego = 0;
ego_lane = RMC.EgoLane;
y_ego = MapInfo.LaneCenters(ego_lane);
numGaps = RMC.NumGaps;
Reachable_matrix = zeros(10, 10);


%%%%%%%%%%%%%%%%%%%%%%%% Make Reachable Matrix %%%%%%%%%%%%%%%%%%%%%%%%%%%%

for i = 1 : numGaps
    for j = 1:numGaps
        if abs(Gaps(i).s - Gaps(j).s) < (Gaps(i).l + Gaps(j).l)/2
            if abs(Gaps(i).lane_idx - Gaps(j).lane_idx) == 1
                Reachable_matrix(i,j) = true;
            else
                Reachable_matrix(i,j) = false;
            end
        else
            Reachable_matrix(i,j) = false;
        end
    end
end

%%%%%%%%%%%%%%%%%%%%%%%%%%% Make Topology %%%%%%%%%%%%%%%%%%%%%%%%%%%%%%%%%

%% root node 정하기
root_node = 0;
for i = 1 : numGaps
    if abs(y_ego - Gaps(i).d) < 0.5
        if (x_ego >= Gaps(i).s - Gaps(i).l/2 ) && (x_ego <= Gaps(i).s + Gaps(i).l/2)
            root_node = Gaps(i).idx;
        end
    end
end

%% edge_list 생성
edge_list = [];
for i = 1 : numGaps
    n = 1;
    for j = 1: numGaps
        if Reachable_matrix(i,j) == 1
            edge_list = [edge_list ; [i,j]];
            Gaps(i).reachable_idx(n) = Gaps(j).idx;
            n = n+1;
        end
    end
end

%% topology 만들기

% root node 추가
S = zeros(1,1);
T = zeros(1,1);
ST = zeros(2, 20);
TS = zeros(2, 20);
eliminate_idx = zeros(1, 10);

for i = 1 : length(edge_list)
    if edge_list(i,1) == root_node
        S = [S root_node];
        T = [T edge_list(i,2)];
    end
end



for i = 1: length(edge_list)
    for j = 1: length(S)
        % Root Node부터 시작해서, Topology 형성
        if edge_list(i,1) == T(j)
            if edge_list(i,2) ~= S(j)
                S = [S edge_list(i,1)];
                T = [T edge_list(i,2)];
            end
        end
    end
end

ST(1:2, 1:length(S)-1) = [S(2:end);T(2:end)];
end

== matlab function SnapshotPlanner/Lane Change Planner/Trajectory Generator/Compute Replanning Signal ==
  data: TrajectoryInfo input; EgoPose input; computeMethod input; TriggerReplan output; timeResolution input
function TriggerReplan  = computeReplanSignal(TrajectoryInfo, EgoPose, computeMethod, timeResolution)
    
    persistent replanTime time

    if isempty(replanTime)
        replanTime = 0;
        time = 0;
    end
    
    if TrajectoryInfo.IsNew
        replanTime = time;
    end
    
    % Initialize output structure
    optimalTrajIndex = TrajectoryInfo.OptimalTrajectoryIndex;
    optimalTrajectory = TrajectoryInfo.GlobalTrajectory(optimalTrajIndex).Trajectory;
    optimalDurationTime = TrajectoryInfo.GlobalTrajectory(optimalTrajIndex).DurationTime;
    numTrajPoints = TrajectoryInfo.GlobalTrajectory(optimalTrajIndex).NumTrajPoints;
    times = TrajectoryInfo.GlobalTrajectory(optimalTrajIndex).Times;
    
    
    % Check StateSelector
    if computeMethod == 1
     
        TriggerReplan = helperComputeReplanTimeBasedOnTime(time,...
                                                           replanTime,...
                                                           numTrajPoints,...
                                                           optimalDurationTime,...
                                                           times,...
                                                           timeResolution);
    
    
    else
        currentPose = [EgoPose.Position(1:2) EgoPose.Yaw];
    
        TriggerReplan = helperComputeReplanTimeBasedOnPose(currentPose, ...
                                                           numTrajPoints, ...
                                                           optimalTrajectory);
    
                                            
    end
    
    time = time + timeResolution;
end

== matlab function SnapshotPlanner/Lane Change Planner/Topology System & Decision Making/Cost Evaluation 1. Road Cost 2. Traffic Cost 3. Arrival Cost 4. Safe Cost 5. Total Cost ==
  data: ST input; globalFrenetStates input; MapInfo input; RMC input Bus: BusRelativeMotionCoordinate; RMC output; target_gap output Bus: BusLaneChangeGap; ego_gap output Bus: BusLaneChangeGap; mioglobaltrajectory input; ego_info output; Mio_info output; EgoBus input
function [RMC, target_gap, ego_gap, ego_info, Mio_info] = CalculateCostFunction(ST, globalFrenetStates, MapInfo, RMC, mioglobaltrajectory, EgoBus)

lane_num = MapInfo.NumLanes;
Num_veh = RMC.veh_number(1:lane_num);
IDs_veh = RMC.veh_Ids(1:sum(Num_veh));
Mio_info = zeros(5, 10);


ego_s = globalFrenetStates.EgoFrenetState(1);
ego_lat = globalFrenetStates.EgoFrenetState(4);
ego_vel_d = globalFrenetStates.EgoFrenetState(5);
ego_acc_d = globalFrenetStates.EgoFrenetState(6);
ego_lane = RMC.EgoLane;

Gaps = RMC.Gaps;
numGaps = RMC.NumGaps;
NumMIOs = mioglobaltrajectory.NumTrajs;
mio_traj = mioglobaltrajectory.Trajectories(1:NumMIOs);
mio_s = zeros(1,NumMIOs);
mio_vel = zeros(1,NumMIOs);
mio_lat = zeros(1,NumMIOs);
mio_ids = zeros(1,NumMIOs);
mio_lane = zeros(1, NumMIOs);

for i = 1:NumMIOs
    mio_s(i) = mio_traj(i).Trajectory(1, 1);
    mio_vel(i) = mio_traj(i).Trajectory(1, 2);
    mio_lat(i) = mio_traj(i).Trajectory(1, 4);
    mio_ids(i) = double(mio_traj(i).TargetID);
    mio_lane(i) = helperDetectLaneNumber(MapInfo, mio_lat(i));
end

mio_info = [mio_s; mio_vel; mio_lat; mio_ids; mio_lane];
Mio_info(1:5,1:NumMIOs) = mio_info;

ego_yaw = -deg2rad(EgoBus.Yaw);
rot_mat = [cos(ego_yaw), -sin(ego_yaw);
           sin(ego_yaw),  cos(ego_yaw)];

ego_vel = rot_mat * [EgoBus.Velocity(1:2)]';
ego_acc = rot_mat * [EgoBus.Acceleration(1:2)]';

ego_vel_s = ego_vel(1);
ego_acc_s = ego_acc(1);


ego_info = [ego_s; ego_vel_s; ego_acc_s; ego_lat; ego_vel_d; ego_acc_d];

Gaps = helperEvaluateRoadCost(numGaps, Gaps);
Gaps = helperEvaluateTrafficCost(numGaps, Gaps, ego_info, MapInfo, mio_info, Num_veh, IDs_veh);
Gaps = helperEvaluateArrivalCost(numGaps, Gaps, ST, MapInfo);
Gaps = helperEvaluateTotalCost(numGaps, Gaps);
RMC.Gaps = Gaps;

s_f = [Gaps.s] + ([Gaps.l]./2);
s_r = [Gaps.s] - ([Gaps.l]./2);
gapidx_ego = 0;
for g = 1:numGaps
    if Gaps(g).d == MapInfo.LaneCenters(ego_lane)
        if s_f(g) >=0
            if s_r(g) <=0
                gapidx_ego = Gaps(g).idx;
            end
        end
    end
end
ego_gap = Gaps(gapidx_ego);

if RMC.veh_number(ego_gap.lane_idx) == 0
    target_gap = ego_gap;
else
    [~, I] = min([Gaps(1:numGaps).total_cost], [], 2, 'omitnan');
    target_gap = Gaps(I(1));
end
end

== matlab function SnapshotPlanner/Lane Change Planner/Trajectory Generator/Compute Current State ==
  data: TrajectoryInfo input; EgoPose input; timestep input; RefPointOnPath output Bus: BusRefPointOnPath; TriggerReplan output
function [RefPointOnPath, TriggerReplan]  = computeCurrentState(TrajectoryInfo,...
                                                                EgoPose, ...
                                                                timestep)
% computeCurrentState estimates the next state of the vehicle based on the
% time or current pose of the ego vehicle.
%
% This function block estimate sthe current pose of the ego vehicle based
% on time or based on current ego pose based on the input from
% StateSelector. If the StateSelector is zero it estimates the pose based
% on current pose, otherwise it estimates state based on time.

persistent replanTime time prev_new 
if isempty(replanTime)
    replanTime = 0;
    time = 0;
    prev_new = false;
end

if (TrajectoryInfo.IsNew && ~prev_new)
    % Time trigger에 의한 궤적이 생성된 경우,
    % Event trigger에 의해 새로운 궤적이 선택된 경우
    replanTime = time;
end

% Initialize output structure
RefPointOnPath = HelperLCPlannerDefaultData.RefPointOnPath;

optimalTrajIndex = TrajectoryInfo.OptimalTrajectoryIndex;
optimalTrajectory = TrajectoryInfo.GlobalTrajectory(optimalTrajIndex).Trajectory;
numTrajPoints = TrajectoryInfo.GlobalTrajectory(optimalTrajIndex).NumTrajPoints;
times = TrajectoryInfo.GlobalTrajectory(optimalTrajIndex).Times;
durationtime = TrajectoryInfo.GlobalTrajectory(optimalTrajIndex).DurationTime;

% Check StateSelector
% Select state based on time
[RefPoseRr,  RefCurvature,...
RefVelocity, RefAccel,...
RefAngVel, RefCurvatureDer,...
LatOffset, RefYawDiff,...
TriggerReplan] = helperComputeCurrentStateBasedOnTime(time,...
                                                      replanTime,...
                                                      numTrajPoints,...
                                                      optimalTrajectory,...
                                                      durationtime,...
                                                      times, ...
                                                      timestep);                                                  

RefPointOnPath.CurrPoseRr       = [EgoPose.Position(1:2) EgoPose.Yaw];
RefPointOnPath.RefPoseRr        = RefPoseRr;
RefPointOnPath.LatOffset        = LatOffset;
RefPointOnPath.RefCurvature     = RefCurvature;
RefPointOnPath.RefCurvatureDer  = RefCurvatureDer;
RefPointOnPath.RefYawDiff       = RefYawDiff;
RefPointOnPath.RefVelocity      = RefVelocity;
RefPointOnPath.RefAccel         = RefAccel;
RefPointOnPath.RefAngVel        = RefAngVel;

time = time + timestep;
prev_new = TrajectoryInfo.IsNew;
end
